simulink model "kalman_estimate_MM"  (R2018b)
settings: Solver=FixedStepAuto  StartTime=0.0  StopTime=500  FixedStep=0.02  RelTol=1e-3
values from neighbouring files (symbols this model uses):
  D = randn(num_output,num_control)    [Com_of_linear_model_calculate.m]    (also in Copy_of_linear_model_calculate.m; D.mat = [0 0 0.00507528406191 0.0236369284061 0.221173094143 0.00198; LINEAR.m = randn(8,1)*10; MM_HKF.m = reshape(out(A_l+B_l+C_l+1:A_l+B_l+C_l+D_l),size_D))
undefined symbols (not defined in the file or in its folder): act_piece, com_piece, piece, sigbuilder_block
libraries: sharedschedule x467, dspsigattribs x44, commchan3 x1
(part 2 of 5)

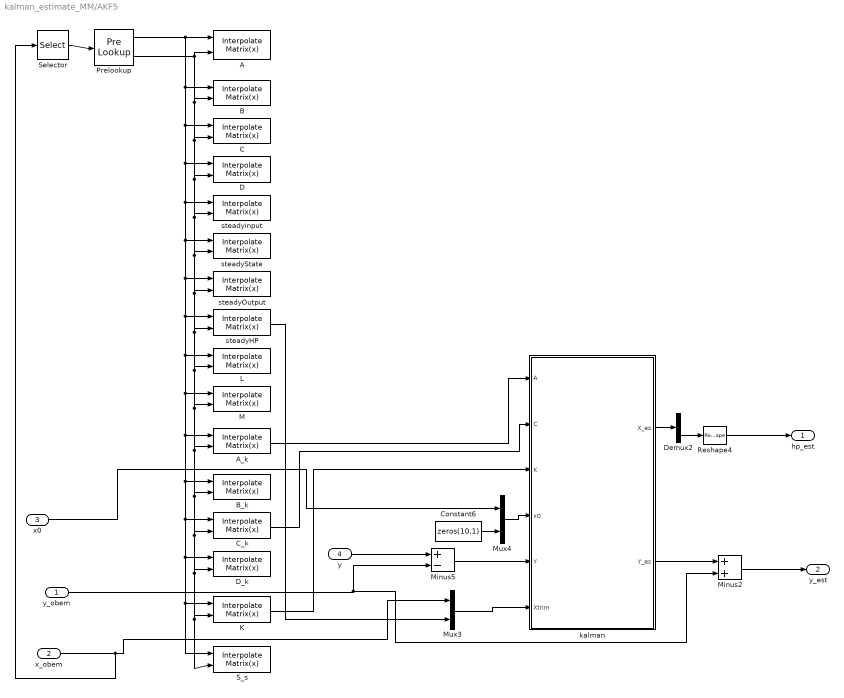
== system kalman_estimate_MM/AKF5 ==
  "y_obem " : Inport
  x_obem : Inport  Port=2
  x0 : Inport  Port=3
  y : Inport  Port=4
  A : sharedschedule/Interpolate Matrix(x)   matrix=piece.A  aMode=aMode
      settings: SourceProductName=Aerospace Blockset  SourceProductBaseCode=AE
  A_k : sharedschedule/Interpolate Matrix(x)   matrix=piece.A_k  aMode=aMode
      settings: SourceProductName=Aerospace Blockset  SourceProductBaseCode=AE
  B : sharedschedule/Interpolate Matrix(x)   matrix=piece.B  aMode=aMode
      settings: SourceProductName=Aerospace Blockset  SourceProductBaseCode=AE
  B_k : sharedschedule/Interpolate Matrix(x)   matrix=piece.B_k  aMode=aMode
      settings: SourceProductName=Aerospace Blockset  SourceProductBaseCode=AE
  C : sharedschedule/Interpolate Matrix(x)   matrix=piece.C  aMode=aMode
      settings: SourceProductName=Aerospace Blockset  SourceProductBaseCode=AE
  C_k : sharedschedule/Interpolate Matrix(x)   matrix=piece.C_k  aMode=aMode
      settings: SourceProductName=Aerospace Blockset  SourceProductBaseCode=AE
  Constant6 : Constant  Value=zeros(10,1)  VectorParams1D=off
  D : sharedschedule/Interpolate Matrix(x)   matrix=piece.D  aMode=aMode
      settings: SourceProductName=Aerospace Blockset  SourceProductBaseCode=AE
  D_k : sharedschedule/Interpolate Matrix(x)   matrix=piece.D_k  aMode=aMode
      settings: SourceProductName=Aerospace Blockset  SourceProductBaseCode=AE
  Demux2 : Demux  Outputs=[2,10]
  K : sharedschedule/Interpolate Matrix(x)   matrix=piece.K  aMode=aMode
      settings: SourceProductName=Aerospace Blockset  SourceProductBaseCode=AE
  L : sharedschedule/Interpolate Matrix(x)   matrix=piece.L  aMode=aMode
      settings: SourceProductName=Aerospace Blockset  SourceProductBaseCode=AE
  M : sharedschedule/Interpolate Matrix(x)   matrix=piece.M  aMode=aMode
      settings: SourceProductName=Aerospace Blockset  SourceProductBaseCode=AE
  Minus2 : Sum
  Minus5 : Sum  Inputs=+-
  Mux3 : Mux  Inputs=2
  Mux4 : Mux  Inputs=2
  Prelookup : PreLookup  BreakpointsData=piece.Nl  BreakpointObject=Nl  ExtrapMethod=Linear  UseLastBreakpoint=on  DiagnosticForOutOfRangeInput=Warning
  Reshape4 : Reshape  OutputDimensionality=Row vector (2-D)
  S_s : sharedschedule/Interpolate Matrix(x)   matrix=piece.K_s  aMode=aMode
      settings: SourceProductName=Aerospace Blockset  SourceProductBaseCode=AE
  Selector : Selector  InputPortWidth=2  IndexOptions=Index vector (dialog)  Indices=[1]  OutputSizes=1
  "kalman " : Subsystem
  steadyHP : sharedschedule/Interpolate Matrix(x)   matrix=piece.steadyHP  aMode=aMode
      settings: SourceProductName=Aerospace Blockset  SourceProductBaseCode=AE
  steadyOutput : sharedschedule/Interpolate Matrix(x)   matrix=piece.steadyOutput  aMode=aMode
      settings: SourceProductName=Aerospace Blockset  SourceProductBaseCode=AE
  steadyState : sharedschedule/Interpolate Matrix(x)   matrix=piece.steadyState  aMode=aMode
      settings: SourceProductName=Aerospace Blockset  SourceProductBaseCode=AE
  steadyinput : sharedschedule/Interpolate Matrix(x)   matrix=piece.steadyInput  aMode=aMode
      settings: SourceProductName=Aerospace Blockset  SourceProductBaseCode=AE
  hp_est : Outport
  y_est : Outport  Port=2
  wires:
  Reshape4/1 -> hp_est/1
  Prelookup/2 -> A/2, S_s/2, K/2, D_k/2, C_k/2, B_k/2, A_k/2, M/2, L/2, steadyHP/2, steadyOutput/2, steadyState/2, steadyinput/2, D/2, C/2, B/2
  Prelookup/1 -> S_s/1, K/1, D_k/1, C_k/1, B_k/1, A_k/1, M/1, L/1, steadyHP/1, steadyOutput/1, steadyState/1, steadyinput/1, D/1, C/1, B/1, A/1
  K/1 -> "kalman "/3(K)
  Selector/1 -> Prelookup/1
  x0/1 -> Mux4/1
  A_k/1 -> "kalman "/1(A)
  "kalman "/1(X_es) -> Demux2/1
  "kalman "/2(Y_es) -> Minus2/1
  Mux3/1 -> "kalman "/6(Xtrim)
  y/1 -> Minus5/1
  Minus5/1 -> "kalman "/5(Y)
  Demux2/2 -> Reshape4/1
  C_k/1 -> "kalman "/2(C)
  "y_obem "/1 -> Minus2/2, Minus5/2
  Mux4/1 -> "kalman "/4(x0)
  Constant6/1 -> Mux4/2
  steadyHP/1 -> Mux3/2
  Minus2/1 -> y_est/1
  x_obem/1 -> Selector/1, Mux3/1

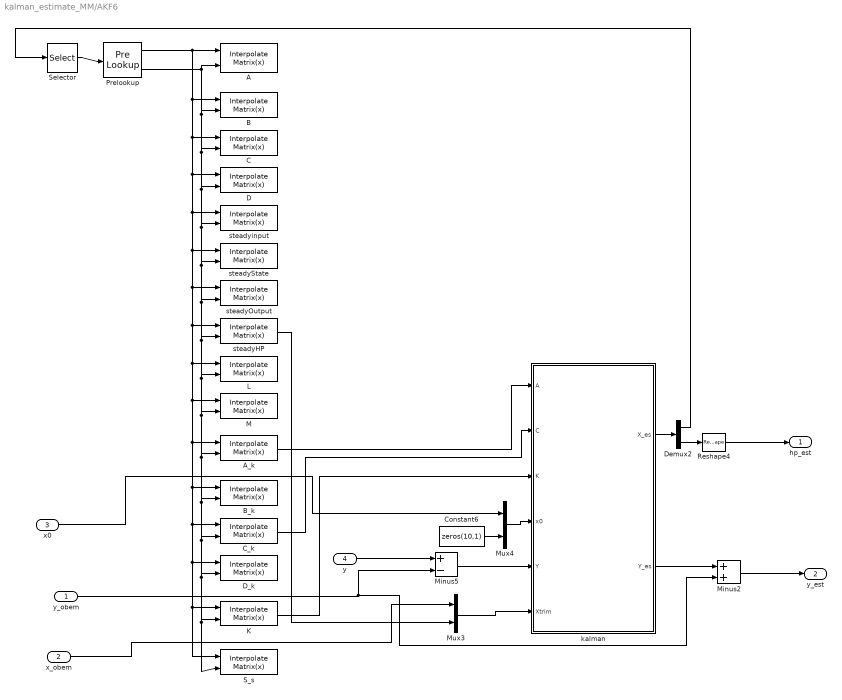
== system kalman_estimate_MM/AKF6 ==
  "y_obem " : Inport
  x_obem : Inport  Port=2
  x0 : Inport  Port=3
  y : Inport  Port=4
  A : sharedschedule/Interpolate Matrix(x)   matrix=piece.A  aMode=aMode
      settings: SourceProductName=Aerospace Blockset  SourceProductBaseCode=AE
  A_k : sharedschedule/Interpolate Matrix(x)   matrix=piece.A_k  aMode=aMode
      settings: SourceProductName=Aerospace Blockset  SourceProductBaseCode=AE
  B : sharedschedule/Interpolate Matrix(x)   matrix=piece.B  aMode=aMode
      settings: SourceProductName=Aerospace Blockset  SourceProductBaseCode=AE
  B_k : sharedschedule/Interpolate Matrix(x)   matrix=piece.B_k  aMode=aMode
      settings: SourceProductName=Aerospace Blockset  SourceProductBaseCode=AE
  C : sharedschedule/Interpolate Matrix(x)   matrix=piece.C  aMode=aMode
      settings: SourceProductName=Aerospace Blockset  SourceProductBaseCode=AE
  C_k : sharedschedule/Interpolate Matrix(x)   matrix=piece.C_k  aMode=aMode
      settings: SourceProductName=Aerospace Blockset  SourceProductBaseCode=AE
  Constant6 : Constant  Value=zeros(10,1)  VectorParams1D=off
  D : sharedschedule/Interpolate Matrix(x)   matrix=piece.D  aMode=aMode
      settings: SourceProductName=Aerospace Blockset  SourceProductBaseCode=AE
  D_k : sharedschedule/Interpolate Matrix(x)   matrix=piece.D_k  aMode=aMode
      settings: SourceProductName=Aerospace Blockset  SourceProductBaseCode=AE
  Demux2 : Demux  Outputs=[2,10]
  K : sharedschedule/Interpolate Matrix(x)   matrix=piece.K  aMode=aMode
      settings: SourceProductName=Aerospace Blockset  SourceProductBaseCode=AE
  L : sharedschedule/Interpolate Matrix(x)   matrix=piece.L  aMode=aMode
      settings: SourceProductName=Aerospace Blockset  SourceProductBaseCode=AE
  M : sharedschedule/Interpolate Matrix(x)   matrix=piece.M  aMode=aMode
      settings: SourceProductName=Aerospace Blockset  SourceProductBaseCode=AE
  Minus2 : Sum
  Minus5 : Sum  Inputs=+-
  Mux3 : Mux  Inputs=2
  Mux4 : Mux  Inputs=2
  Prelookup : PreLookup  BreakpointsData=piece.Nl  BreakpointObject=Nl  ExtrapMethod=Linear  UseLastBreakpoint=on  DiagnosticForOutOfRangeInput=Warning
  Reshape4 : Reshape  OutputDimensionality=Row vector (2-D)
  S_s : sharedschedule/Interpolate Matrix(x)   matrix=piece.K_s  aMode=aMode
      settings: SourceProductName=Aerospace Blockset  SourceProductBaseCode=AE
  Selector : Selector  InputPortWidth=2  IndexOptions=Index vector (dialog)  Indices=[1]  OutputSizes=1
  "kalman " : Subsystem
  steadyHP : sharedschedule/Interpolate Matrix(x)   matrix=piece.steadyHP  aMode=aMode
      settings: SourceProductName=Aerospace Blockset  SourceProductBaseCode=AE
  steadyOutput : sharedschedule/Interpolate Matrix(x)   matrix=piece.steadyOutput  aMode=aMode
      settings: SourceProductName=Aerospace Blockset  SourceProductBaseCode=AE
  steadyState : sharedschedule/Interpolate Matrix(x)   matrix=piece.steadyState  aMode=aMode
      settings: SourceProductName=Aerospace Blockset  SourceProductBaseCode=AE
  steadyinput : sharedschedule/Interpolate Matrix(x)   matrix=piece.steadyInput  aMode=aMode
      settings: SourceProductName=Aerospace Blockset  SourceProductBaseCode=AE
  hp_est : Outport
  y_est : Outport  Port=2
  wires:
  x_obem/1 -> Mux3/1
  Minus2/1 -> y_est/1
  steadyHP/1 -> Mux3/2
  Constant6/1 -> Mux4/2
  Mux4/1 -> "kalman "/4(x0)
  "y_obem "/1 -> Minus5/2, Minus2/2
  C_k/1 -> "kalman "/2(C)
  Demux2/2 -> Reshape4/1
  Minus5/1 -> "kalman "/5(Y)
  y/1 -> Minus5/1
  Mux3/1 -> "kalman "/6(Xtrim)
  "kalman "/2(Y_es) -> Minus2/1
  Demux2/1 -> Selector/1
  "kalman "/1(X_es) -> Demux2/1
  A_k/1 -> "kalman "/1(A)
  x0/1 -> Mux4/1
  Selector/1 -> Prelookup/1
  K/1 -> "kalman "/3(K)
  Prelookup/1 -> A/1, B/1, C/1, D/1, steadyinput/1, steadyState/1, steadyOutput/1, steadyHP/1, L/1, M/1, A_k/1, B_k/1, C_k/1, D_k/1, K/1, S_s/1
  Prelookup/2 -> B/2, C/2, D/2, steadyinput/2, steadyState/2, steadyOutput/2, steadyHP/2, L/2, M/2, A_k/2, B_k/2, C_k/2, D_k/2, K/2, S_s/2, A/2
  Reshape4/1 -> hp_est/1

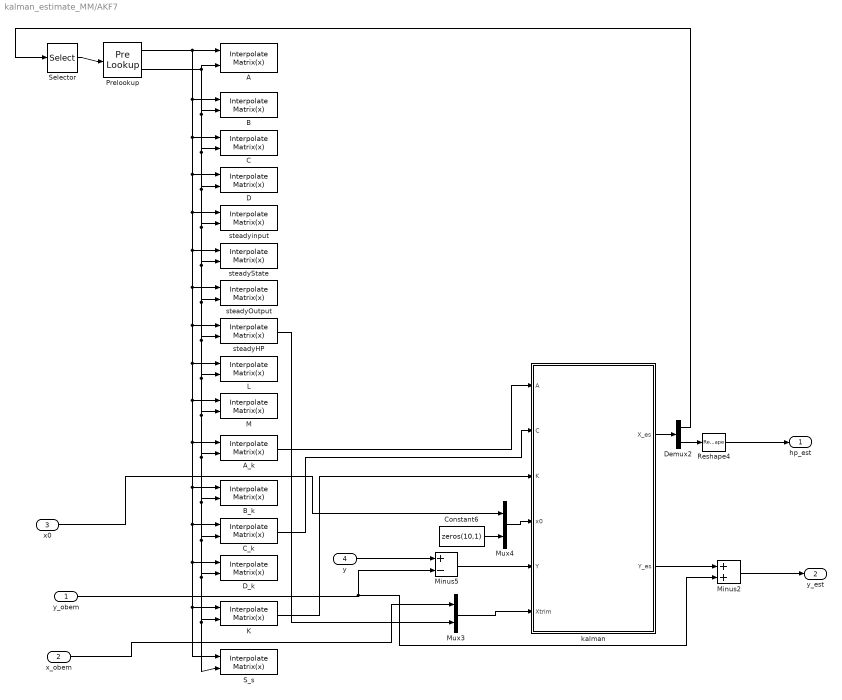
== system kalman_estimate_MM/AKF7 ==
  "y_obem " : Inport
  x_obem : Inport  Port=2
  x0 : Inport  Port=3
  y : Inport  Port=4
  A : sharedschedule/Interpolate Matrix(x)   matrix=piece.A  aMode=aMode
      settings: SourceProductName=Aerospace Blockset  SourceProductBaseCode=AE
  A_k : sharedschedule/Interpolate Matrix(x)   matrix=piece.A_k  aMode=aMode
      settings: SourceProductName=Aerospace Blockset  SourceProductBaseCode=AE
  B : sharedschedule/Interpolate Matrix(x)   matrix=piece.B  aMode=aMode
      settings: SourceProductName=Aerospace Blockset  SourceProductBaseCode=AE
  B_k : sharedschedule/Interpolate Matrix(x)   matrix=piece.B_k  aMode=aMode
      settings: SourceProductName=Aerospace Blockset  SourceProductBaseCode=AE
  C : sharedschedule/Interpolate Matrix(x)   matrix=piece.C  aMode=aMode
      settings: SourceProductName=Aerospace Blockset  SourceProductBaseCode=AE
  C_k : sharedschedule/Interpolate Matrix(x)   matrix=piece.C_k  aMode=aMode
      settings: SourceProductName=Aerospace Blockset  SourceProductBaseCode=AE
  Constant6 : Constant  Value=zeros(10,1)  VectorParams1D=off
  D : sharedschedule/Interpolate Matrix(x)   matrix=piece.D  aMode=aMode
      settings: SourceProductName=Aerospace Blockset  SourceProductBaseCode=AE
  D_k : sharedschedule/Interpolate Matrix(x)   matrix=piece.D_k  aMode=aMode
      settings: SourceProductName=Aerospace Blockset  SourceProductBaseCode=AE
  Demux2 : Demux  Outputs=[2,10]
  K : sharedschedule/Interpolate Matrix(x)   matrix=piece.K  aMode=aMode
      settings: SourceProductName=Aerospace Blockset  SourceProductBaseCode=AE
  L : sharedschedule/Interpolate Matrix(x)   matrix=piece.L  aMode=aMode
      settings: SourceProductName=Aerospace Blockset  SourceProductBaseCode=AE
  M : sharedschedule/Interpolate Matrix(x)   matrix=piece.M  aMode=aMode
      settings: SourceProductName=Aerospace Blockset  SourceProductBaseCode=AE
  Minus2 : Sum
  Minus5 : Sum  Inputs=+-
  Mux3 : Mux  Inputs=2
  Mux4 : Mux  Inputs=2
  Prelookup : PreLookup  BreakpointsData=piece.Nl  BreakpointObject=Nl  ExtrapMethod=Linear  UseLastBreakpoint=on  DiagnosticForOutOfRangeInput=Warning
  Reshape4 : Reshape  OutputDimensionality=Row vector (2-D)
  S_s : sharedschedule/Interpolate Matrix(x)   matrix=piece.K_s  aMode=aMode
      settings: SourceProductName=Aerospace Blockset  SourceProductBaseCode=AE
  Selector : Selector  InputPortWidth=2  IndexOptions=Index vector (dialog)  Indices=[1]  OutputSizes=1
  "kalman " : Subsystem
  steadyHP : sharedschedule/Interpolate Matrix(x)   matrix=piece.steadyHP  aMode=aMode
      settings: SourceProductName=Aerospace Blockset  SourceProductBaseCode=AE
  steadyOutput : sharedschedule/Interpolate Matrix(x)   matrix=piece.steadyOutput  aMode=aMode
      settings: SourceProductName=Aerospace Blockset  SourceProductBaseCode=AE
  steadyState : sharedschedule/Interpolate Matrix(x)   matrix=piece.steadyState  aMode=aMode
      settings: SourceProductName=Aerospace Blockset  SourceProductBaseCode=AE
  steadyinput : sharedschedule/Interpolate Matrix(x)   matrix=piece.steadyInput  aMode=aMode
      settings: SourceProductName=Aerospace Blockset  SourceProductBaseCode=AE
  hp_est : Outport
  y_est : Outport  Port=2
  wires:
  Reshape4/1 -> hp_est/1
  Prelookup/2 -> A/2, S_s/2, K/2, D_k/2, C_k/2, B_k/2, A_k/2, M/2, L/2, steadyHP/2, steadyOutput/2, steadyState/2, steadyinput/2, D/2, C/2, B/2
  Prelookup/1 -> S_s/1, K/1, D_k/1, C_k/1, B_k/1, A_k/1, M/1, L/1, steadyHP/1, steadyOutput/1, steadyState/1, steadyinput/1, D/1, C/1, B/1, A/1
  K/1 -> "kalman "/3(K)
  Selector/1 -> Prelookup/1
  x0/1 -> Mux4/1
  A_k/1 -> "kalman "/1(A)
  "kalman "/1(X_es) -> Demux2/1
  Demux2/1 -> Selector/1
  "kalman "/2(Y_es) -> Minus2/1
  Mux3/1 -> "kalman "/6(Xtrim)
  y/1 -> Minus5/1
  Minus5/1 -> "kalman "/5(Y)
  Demux2/2 -> Reshape4/1
  C_k/1 -> "kalman "/2(C)
  "y_obem "/1 -> Minus2/2, Minus5/2
  Mux4/1 -> "kalman "/4(x0)
  Constant6/1 -> Mux4/2
  steadyHP/1 -> Mux3/2
  Minus2/1 -> y_est/1
  x_obem/1 -> Mux3/1

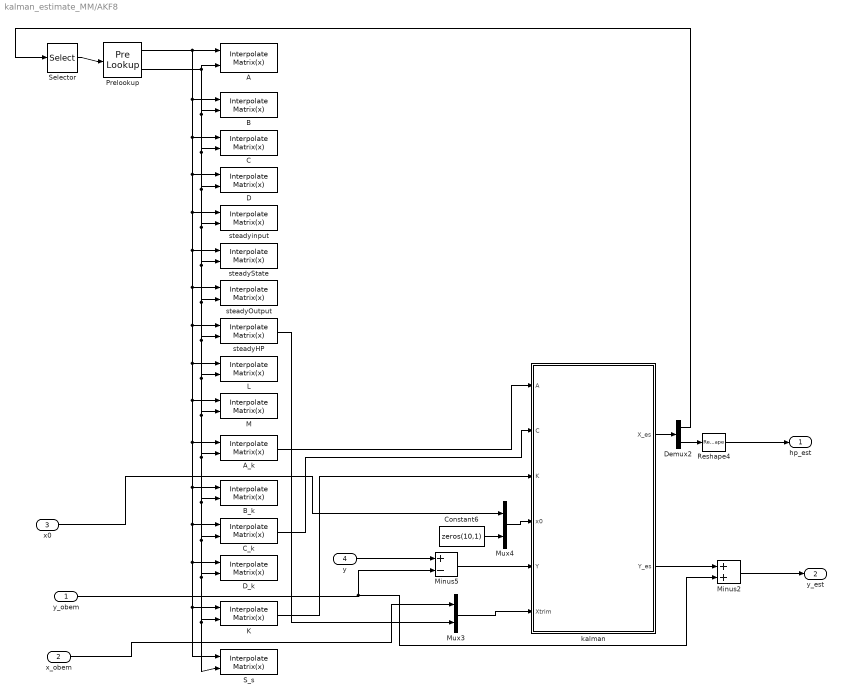
== system kalman_estimate_MM/AKF8 ==
  "y_obem " : Inport
  x_obem : Inport  Port=2
  x0 : Inport  Port=3
  y : Inport  Port=4
  A : sharedschedule/Interpolate Matrix(x)   matrix=piece.A  aMode=aMode
      settings: SourceProductName=Aerospace Blockset  SourceProductBaseCode=AE
  A_k : sharedschedule/Interpolate Matrix(x)   matrix=piece.A_k  aMode=aMode
      settings: SourceProductName=Aerospace Blockset  SourceProductBaseCode=AE
  B : sharedschedule/Interpolate Matrix(x)   matrix=piece.B  aMode=aMode
      settings: SourceProductName=Aerospace Blockset  SourceProductBaseCode=AE
  B_k : sharedschedule/Interpolate Matrix(x)   matrix=piece.B_k  aMode=aMode
      settings: SourceProductName=Aerospace Blockset  SourceProductBaseCode=AE
  C : sharedschedule/Interpolate Matrix(x)   matrix=piece.C  aMode=aMode
      settings: SourceProductName=Aerospace Blockset  SourceProductBaseCode=AE
  C_k : sharedschedule/Interpolate Matrix(x)   matrix=piece.C_k  aMode=aMode
      settings: SourceProductName=Aerospace Blockset  SourceProductBaseCode=AE
  Constant6 : Constant  Value=zeros(10,1)  VectorParams1D=off
  D : sharedschedule/Interpolate Matrix(x)   matrix=piece.D  aMode=aMode
      settings: SourceProductName=Aerospace Blockset  SourceProductBaseCode=AE
  D_k : sharedschedule/Interpolate Matrix(x)   matrix=piece.D_k  aMode=aMode
      settings: SourceProductName=Aerospace Blockset  SourceProductBaseCode=AE
  Demux2 : Demux  Outputs=[2,10]
  K : sharedschedule/Interpolate Matrix(x)   matrix=piece.K  aMode=aMode
      settings: SourceProductName=Aerospace Blockset  SourceProductBaseCode=AE
  L : sharedschedule/Interpolate Matrix(x)   matrix=piece.L  aMode=aMode
      settings: SourceProductName=Aerospace Blockset  SourceProductBaseCode=AE
  M : sharedschedule/Interpolate Matrix(x)   matrix=piece.M  aMode=aMode
      settings: SourceProductName=Aerospace Blockset  SourceProductBaseCode=AE
  Minus2 : Sum
  Minus5 : Sum  Inputs=+-
  Mux3 : Mux  Inputs=2
  Mux4 : Mux  Inputs=2
  Prelookup : PreLookup  BreakpointsData=piece.Nl  BreakpointObject=Nl  ExtrapMethod=Linear  UseLastBreakpoint=on  DiagnosticForOutOfRangeInput=Warning
  Reshape4 : Reshape  OutputDimensionality=Row vector (2-D)
  S_s : sharedschedule/Interpolate Matrix(x)   matrix=piece.K_s  aMode=aMode
      settings: SourceProductName=Aerospace Blockset  SourceProductBaseCode=AE
  Selector : Selector  InputPortWidth=2  IndexOptions=Index vector (dialog)  Indices=[1]  OutputSizes=1
  "kalman " : Subsystem
  steadyHP : sharedschedule/Interpolate Matrix(x)   matrix=piece.steadyHP  aMode=aMode
      settings: SourceProductName=Aerospace Blockset  SourceProductBaseCode=AE
  steadyOutput : sharedschedule/Interpolate Matrix(x)   matrix=piece.steadyOutput  aMode=aMode
      settings: SourceProductName=Aerospace Blockset  SourceProductBaseCode=AE
  steadyState : sharedschedule/Interpolate Matrix(x)   matrix=piece.steadyState  aMode=aMode
      settings: SourceProductName=Aerospace Blockset  SourceProductBaseCode=AE
  steadyinput : sharedschedule/Interpolate Matrix(x)   matrix=piece.steadyInput  aMode=aMode
      settings: SourceProductName=Aerospace Blockset  SourceProductBaseCode=AE
  hp_est : Outport
  y_est : Outport  Port=2
  wires:
  x_obem/1 -> Mux3/1
  Minus2/1 -> y_est/1
  steadyHP/1 -> Mux3/2
  Constant6/1 -> Mux4/2
  Mux4/1 -> "kalman "/4(x0)
  "y_obem "/1 -> Minus5/2, Minus2/2
  C_k/1 -> "kalman "/2(C)
  Demux2/2 -> Reshape4/1
  Minus5/1 -> "kalman "/5(Y)
  y/1 -> Minus5/1
  Mux3/1 -> "kalman "/6(Xtrim)
  "kalman "/2(Y_es) -> Minus2/1
  Demux2/1 -> Selector/1
  "kalman "/1(X_es) -> Demux2/1
  A_k/1 -> "kalman "/1(A)
  x0/1 -> Mux4/1
  Selector/1 -> Prelookup/1
  K/1 -> "kalman "/3(K)
  Prelookup/1 -> A/1, B/1, C/1, D/1, steadyinput/1, steadyState/1, steadyOutput/1, steadyHP/1, L/1, M/1, A_k/1, B_k/1, C_k/1, D_k/1, K/1, S_s/1
  Prelookup/2 -> B/2, C/2, D/2, steadyinput/2, steadyState/2, steadyOutput/2, steadyHP/2, L/2, M/2, A_k/2, B_k/2, C_k/2, D_k/2, K/2, S_s/2, A/2
  Reshape4/1 -> hp_est/1

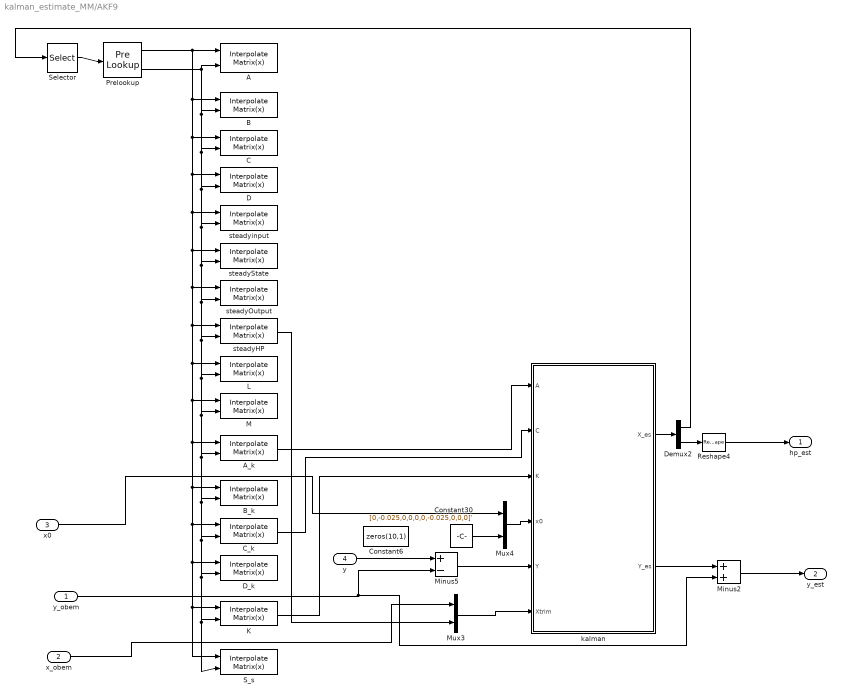
== system kalman_estimate_MM/AKF9 ==
  "y_obem " : Inport
  x_obem : Inport  Port=2
  x0 : Inport  Port=3
  y : Inport  Port=4
  A : sharedschedule/Interpolate Matrix(x)   matrix=piece.A  aMode=aMode
      settings: SourceProductName=Aerospace Blockset  SourceProductBaseCode=AE
  A_k : sharedschedule/Interpolate Matrix(x)   matrix=piece.A_k  aMode=aMode
      settings: SourceProductName=Aerospace Blockset  SourceProductBaseCode=AE
  B : sharedschedule/Interpolate Matrix(x)   matrix=piece.B  aMode=aMode
      settings: SourceProductName=Aerospace Blockset  SourceProductBaseCode=AE
  B_k : sharedschedule/Interpolate Matrix(x)   matrix=piece.B_k  aMode=aMode
      settings: SourceProductName=Aerospace Blockset  SourceProductBaseCode=AE
  C : sharedschedule/Interpolate Matrix(x)   matrix=piece.C  aMode=aMode
      settings: SourceProductName=Aerospace Blockset  SourceProductBaseCode=AE
  C_k : sharedschedule/Interpolate Matrix(x)   matrix=piece.C_k  aMode=aMode
      settings: SourceProductName=Aerospace Blockset  SourceProductBaseCode=AE
  Constant30 : Constant  Value=[0,-0.025,0,0,0,0,-0.025,0,0,0]'  VectorParams1D=off
  Constant6 : Constant  Value=zeros(10,1)  VectorParams1D=off
  D : sharedschedule/Interpolate Matrix(x)   matrix=piece.D  aMode=aMode
      settings: SourceProductName=Aerospace Blockset  SourceProductBaseCode=AE
  D_k : sharedschedule/Interpolate Matrix(x)   matrix=piece.D_k  aMode=aMode
      settings: SourceProductName=Aerospace Blockset  SourceProductBaseCode=AE
  Demux2 : Demux  Outputs=[2,10]
  K : sharedschedule/Interpolate Matrix(x)   matrix=piece.K  aMode=aMode
      settings: SourceProductName=Aerospace Blockset  SourceProductBaseCode=AE
  L : sharedschedule/Interpolate Matrix(x)   matrix=piece.L  aMode=aMode
      settings: SourceProductName=Aerospace Blockset  SourceProductBaseCode=AE
  M : sharedschedule/Interpolate Matrix(x)   matrix=piece.M  aMode=aMode
      settings: SourceProductName=Aerospace Blockset  SourceProductBaseCode=AE
  Minus2 : Sum
  Minus5 : Sum  Inputs=+-
  Mux3 : Mux  Inputs=2
  Mux4 : Mux  Inputs=2
  Prelookup : PreLookup  BreakpointsData=piece.Nl  BreakpointObject=Nl  ExtrapMethod=Linear  UseLastBreakpoint=on  DiagnosticForOutOfRangeInput=Warning
  Reshape4 : Reshape  OutputDimensionality=Row vector (2-D)
  S_s : sharedschedule/Interpolate Matrix(x)   matrix=piece.K_s  aMode=aMode
      settings: SourceProductName=Aerospace Blockset  SourceProductBaseCode=AE
  Selector : Selector  InputPortWidth=2  IndexOptions=Index vector (dialog)  Indices=[1]  OutputSizes=1
  "kalman " : Subsystem
  steadyHP : sharedschedule/Interpolate Matrix(x)   matrix=piece.steadyHP  aMode=aMode
      settings: SourceProductName=Aerospace Blockset  SourceProductBaseCode=AE
  steadyOutput : sharedschedule/Interpolate Matrix(x)   matrix=piece.steadyOutput  aMode=aMode
      settings: SourceProductName=Aerospace Blockset  SourceProductBaseCode=AE
  steadyState : sharedschedule/Interpolate Matrix(x)   matrix=piece.steadyState  aMode=aMode
      settings: SourceProductName=Aerospace Blockset  SourceProductBaseCode=AE
  steadyinput : sharedschedule/Interpolate Matrix(x)   matrix=piece.steadyInput  aMode=aMode
      settings: SourceProductName=Aerospace Blockset  SourceProductBaseCode=AE
  hp_est : Outport
  y_est : Outport  Port=2
  wires:
  Reshape4/1 -> hp_est/1
  Prelookup/2 -> A/2, S_s/2, K/2, D_k/2, C_k/2, B_k/2, A_k/2, M/2, L/2, steadyHP/2, steadyOutput/2, steadyState/2, steadyinput/2, D/2, C/2, B/2
  Prelookup/1 -> S_s/1, K/1, D_k/1, C_k/1, B_k/1, A_k/1, M/1, L/1, steadyHP/1, steadyOutput/1, steadyState/1, steadyinput/1, D/1, C/1, B/1, A/1
  K/1 -> "kalman "/3(K)
  Selector/1 -> Prelookup/1
  x0/1 -> Mux4/1
  A_k/1 -> "kalman "/1(A)
  "kalman "/1(X_es) -> Demux2/1
  Demux2/1 -> Selector/1
  "kalman "/2(Y_es) -> Minus2/1
  Mux3/1 -> "kalman "/6(Xtrim)
  y/1 -> Minus5/1
  Minus5/1 -> "kalman "/5(Y)
  Demux2/2 -> Reshape4/1
  C_k/1 -> "kalman "/2(C)
  "y_obem "/1 -> Minus2/2, Minus5/2
  Mux4/1 -> "kalman "/4(x0)
  steadyHP/1 -> Mux3/2
  Minus2/1 -> y_est/1
  x_obem/1 -> Mux3/1
  Constant30/1 -> Mux4/2

== system kalman_estimate_MM/HKF1 ==
  In2 : Inport
  In3 : Inport  Port=2
  In4 : Inport  Port=3
  x_obem : Inport  Port=4
  y_obem : Inport  Port=5
  A : sharedschedule/Interpolate Matrix(x)   matrix=piece.A  aMode=aMode
      settings: SourceProductName=Aerospace Blockset  SourceProductBaseCode=AE
  B : sharedschedule/Interpolate Matrix(x)   matrix=piece.B  aMode=aMode
      settings: SourceProductName=Aerospace Blockset  SourceProductBaseCode=AE
  C : sharedschedule/Interpolate Matrix(x)   matrix=piece.C  aMode=aMode
      settings: SourceProductName=Aerospace Blockset  SourceProductBaseCode=AE
  D : sharedschedule/Interpolate Matrix(x)   matrix=piece.D  aMode=aMode
      settings: SourceProductName=Aerospace Blockset  SourceProductBaseCode=AE
  K_s : sharedschedule/Interpolate Matrix(x)   matrix=piece.K_s  aMode=aMode
      settings: SourceProductName=Aerospace Blockset  SourceProductBaseCode=AE
  L : sharedschedule/Interpolate Matrix(x)   matrix=piece.L  aMode=aMode
      settings: SourceProductName=Aerospace Blockset  SourceProductBaseCode=AE
  M : sharedschedule/Interpolate Matrix(x)   matrix=piece.M  aMode=aMode
      settings: SourceProductName=Aerospace Blockset  SourceProductBaseCode=AE
  MATLAB Function : MATLAB Function  TreatAsAtomicUnit=on
  Minus5 : Sum  Inputs=+-
  Prelookup : PreLookup  BreakpointsData=piece.Nl  BreakpointObject=Nl  ExtrapMethod=Linear  UseLastBreakpoint=on  DiagnosticForOutOfRangeInput=Warning
  S : sharedschedule/Interpolate Matrix(x)   matrix=piece.S_s  aMode=aMode
      settings: SourceProductName=Aerospace Blockset  SourceProductBaseCode=AE
  Selector : Selector  InputPortWidth=2  IndexOptions=Index vector (dialog)  Indices=[1]  OutputSizes=1
  kalman filter1 : Subsystem
  steadyOutput : sharedschedule/Interpolate Matrix(x)   matrix=piece.steadyOutput  aMode=aMode
      settings: SourceProductName=Aerospace Blockset  SourceProductBaseCode=AE
  steadyState : sharedschedule/Interpolate Matrix(x)   matrix=piece.steadyState  aMode=aMode
      settings: SourceProductName=Aerospace Blockset  SourceProductBaseCode=AE
  steadyinput : sharedschedule/Interpolate Matrix(x)   matrix=piece.steadyInput  aMode=aMode
      settings: SourceProductName=Aerospace Blockset  SourceProductBaseCode=AE
  Out1 : Outport
  Out2 : Outport  Port=2
  Out3 : Outport  Port=3
  wires:
  x_obem/1 -> kalman filter1/6(Xtrim)
  y_obem/1 -> Minus5/2
  In2/1 -> Minus5/1
  In3/1 -> kalman filter1/4(x0)
  M/1 -> kalman filter1/8(M)
  A/1 -> kalman filter1/1(A)
  K_s/1 -> kalman filter1/3(K)
  kalman filter1/1(X_es) -> Selector/1
  kalman filter1/2(Y_es) -> Out1/1
  Minus5/1 -> kalman filter1/5(Y)
  C/1 -> kalman filter1/2(C)
  L/1 -> kalman filter1/7(L)
  Selector/1 -> Prelookup/1
  Prelookup/2 -> B/2, C/2, D/2, steadyOutput/2, steadyinput/2, L/2, M/2, K_s/2, S/2, steadyState/2, A/2
  In4/1 -> kalman filter1/9(P)
  Prelookup/1 -> A/1, B/1, C/1, D/1, steadyOutput/1, steadyinput/1, steadyState/1, L/1, M/1, K_s/1, S/1
  MATLAB Function/1(y) -> Out3/1
  kalman filter1/3(Y_error) -> MATLAB Function/1(err), Out2/1
  S/1 -> MATLAB Function/2(S)

== system kalman_estimate_MM/HKF10 ==
  In3 : Inport
  In4 : Inport  Port=2
  x_obem : Inport  Port=3
  y_obem : Inport  Port=4
  A : sharedschedule/Interpolate Matrix(x)   matrix=piece.A  aMode=aMode
      settings: SourceProductName=Aerospace Blockset  SourceProductBaseCode=AE
  Add : Sum
  B : sharedschedule/Interpolate Matrix(x)   matrix=piece.B  aMode=aMode
      settings: SourceProductName=Aerospace Blockset  SourceProductBaseCode=AE
  C : sharedschedule/Interpolate Matrix(x)   matrix=piece.C  aMode=aMode
      settings: SourceProductName=Aerospace Blockset  SourceProductBaseCode=AE
  D : sharedschedule/Interpolate Matrix(x)   matrix=piece.D  aMode=aMode
      settings: SourceProductName=Aerospace Blockset  SourceProductBaseCode=AE
  K_s : sharedschedule/Interpolate Matrix(x)   matrix=piece.K_s  aMode=aMode
      settings: SourceProductName=Aerospace Blockset  SourceProductBaseCode=AE
  L : sharedschedule/Interpolate Matrix(x)   matrix=piece.L  aMode=aMode
      settings: SourceProductName=Aerospace Blockset  SourceProductBaseCode=AE
  M : sharedschedule/Interpolate Matrix(x)   matrix=piece.M  aMode=aMode
      settings: SourceProductName=Aerospace Blockset  SourceProductBaseCode=AE
  Prelookup : PreLookup  BreakpointsData=piece.Nl  BreakpointObject=Nl  ExtrapMethod=Linear  UseLastBreakpoint=on  DiagnosticForOutOfRangeInput=Warning
  S : sharedschedule/Interpolate Matrix(x)   matrix=piece.S_s  aMode=aMode
      settings: SourceProductName=Aerospace Blockset  SourceProductBaseCode=AE
  Selector : Selector  InputPortWidth=2  IndexOptions=Index vector (dialog)  Indices=[1]  OutputSizes=1
  kalman filter1 : Subsystem
  steadyOutput : sharedschedule/Interpolate Matrix(x)   matrix=piece.steadyOutput  aMode=aMode
      settings: SourceProductName=Aerospace Blockset  SourceProductBaseCode=AE
  steadyState : sharedschedule/Interpolate Matrix(x)   matrix=piece.steadyState  aMode=aMode
      settings: SourceProductName=Aerospace Blockset  SourceProductBaseCode=AE
  steadyinput : sharedschedule/Interpolate Matrix(x)   matrix=piece.steadyInput  aMode=aMode
      settings: SourceProductName=Aerospace Blockset  SourceProductBaseCode=AE
  Out1 : Outport
  Out2 : Outport  Port=2
  wires:
  Prelookup/1 -> S/1, K_s/1, M/1, L/1, steadyState/1, steadyinput/1, steadyOutput/1, D/1, C/1, B/1, A/1
  In4/1 -> kalman filter1/7(P)
  Prelookup/2 -> A/2, steadyState/2, S/2, K_s/2, M/2, L/2, steadyinput/2, steadyOutput/2, D/2, C/2, B/2
  Selector/1 -> Prelookup/1
  L/1 -> kalman filter1/5(L)
  C/1 -> kalman filter1/2(C)
  kalman filter1/1(X_es) -> Selector/1
  A/1 -> kalman filter1/1(A)
  M/1 -> kalman filter1/6(M)
  In3/1 -> kalman filter1/3(x0)
  x_obem/1 -> kalman filter1/4(Xtrim)
  y_obem/1 -> Add/2
  kalman filter1/2(Y_es) -> Add/1, Out1/1
  Add/1 -> Out2/1

== system kalman_estimate_MM/HKF11 ==
  In3 : Inport
  In4 : Inport  Port=2
  x_obem : Inport  Port=3
  y_obem : Inport  Port=4
  A : sharedschedule/Interpolate Matrix(x)   matrix=piece.A  aMode=aMode
      settings: SourceProductName=Aerospace Blockset  SourceProductBaseCode=AE
  Add : Sum
  B : sharedschedule/Interpolate Matrix(x)   matrix=piece.B  aMode=aMode
      settings: SourceProductName=Aerospace Blockset  SourceProductBaseCode=AE
  C : sharedschedule/Interpolate Matrix(x)   matrix=piece.C  aMode=aMode
      settings: SourceProductName=Aerospace Blockset  SourceProductBaseCode=AE
  D : sharedschedule/Interpolate Matrix(x)   matrix=piece.D  aMode=aMode
      settings: SourceProductName=Aerospace Blockset  SourceProductBaseCode=AE
  K_s : sharedschedule/Interpolate Matrix(x)   matrix=piece.K_s  aMode=aMode
      settings: SourceProductName=Aerospace Blockset  SourceProductBaseCode=AE
  L : sharedschedule/Interpolate Matrix(x)   matrix=piece.L  aMode=aMode
      settings: SourceProductName=Aerospace Blockset  SourceProductBaseCode=AE
  M : sharedschedule/Interpolate Matrix(x)   matrix=piece.M  aMode=aMode
      settings: SourceProductName=Aerospace Blockset  SourceProductBaseCode=AE
  Prelookup : PreLookup  BreakpointsData=piece.Nl  BreakpointObject=Nl  ExtrapMethod=Linear  UseLastBreakpoint=on  DiagnosticForOutOfRangeInput=Warning
  S : sharedschedule/Interpolate Matrix(x)   matrix=piece.S_s  aMode=aMode
      settings: SourceProductName=Aerospace Blockset  SourceProductBaseCode=AE
  Selector : Selector  InputPortWidth=2  IndexOptions=Index vector (dialog)  Indices=[1]  OutputSizes=1
  kalman filter1 : Subsystem
  steadyOutput : sharedschedule/Interpolate Matrix(x)   matrix=piece.steadyOutput  aMode=aMode
      settings: SourceProductName=Aerospace Blockset  SourceProductBaseCode=AE
  steadyState : sharedschedule/Interpolate Matrix(x)   matrix=piece.steadyState  aMode=aMode
      settings: SourceProductName=Aerospace Blockset  SourceProductBaseCode=AE
  steadyinput : sharedschedule/Interpolate Matrix(x)   matrix=piece.steadyInput  aMode=aMode
      settings: SourceProductName=Aerospace Blockset  SourceProductBaseCode=AE
  Out1 : Outport
  Out2 : Outport  Port=2
  wires:
  Add/1 -> Out2/1
  kalman filter1/2(Y_es) -> Out1/1, Add/1
  y_obem/1 -> Add/2
  x_obem/1 -> kalman filter1/4(Xtrim)
  In3/1 -> kalman filter1/3(x0)
  M/1 -> kalman filter1/6(M)
  A/1 -> kalman filter1/1(A)
  kalman filter1/1(X_es) -> Selector/1
  C/1 -> kalman filter1/2(C)
  L/1 -> kalman filter1/5(L)
  Selector/1 -> Prelookup/1
  Prelookup/2 -> B/2, C/2, D/2, steadyOutput/2, steadyinput/2, L/2, M/2, K_s/2, S/2, steadyState/2, A/2
  In4/1 -> kalman filter1/7(P)
  Prelookup/1 -> A/1, B/1, C/1, D/1, steadyOutput/1, steadyinput/1, steadyState/1, L/1, M/1, K_s/1, S/1

== system kalman_estimate_MM/HKF2 ==
  In3 : Inport
  In4 : Inport  Port=2
  x_obem : Inport  Port=3
  y_obem : Inport  Port=4
  A : sharedschedule/Interpolate Matrix(x)   matrix=piece.A  aMode=aMode
      settings: SourceProductName=Aerospace Blockset  SourceProductBaseCode=AE
  Add : Sum
  B : sharedschedule/Interpolate Matrix(x)   matrix=piece.B  aMode=aMode
      settings: SourceProductName=Aerospace Blockset  SourceProductBaseCode=AE
  C : sharedschedule/Interpolate Matrix(x)   matrix=piece.C  aMode=aMode
      settings: SourceProductName=Aerospace Blockset  SourceProductBaseCode=AE
  D : sharedschedule/Interpolate Matrix(x)   matrix=piece.D  aMode=aMode
      settings: SourceProductName=Aerospace Blockset  SourceProductBaseCode=AE
  K_s : sharedschedule/Interpolate Matrix(x)   matrix=piece.K_s  aMode=aMode
      settings: SourceProductName=Aerospace Blockset  SourceProductBaseCode=AE
  L : sharedschedule/Interpolate Matrix(x)   matrix=piece.L  aMode=aMode
      settings: SourceProductName=Aerospace Blockset  SourceProductBaseCode=AE
  M : sharedschedule/Interpolate Matrix(x)   matrix=piece.M  aMode=aMode
      settings: SourceProductName=Aerospace Blockset  SourceProductBaseCode=AE
  Prelookup : PreLookup  BreakpointsData=piece.Nl  BreakpointObject=Nl  ExtrapMethod=Linear  UseLastBreakpoint=on  DiagnosticForOutOfRangeInput=Warning
  S : sharedschedule/Interpolate Matrix(x)   matrix=piece.S_s  aMode=aMode
      settings: SourceProductName=Aerospace Blockset  SourceProductBaseCode=AE
  Selector : Selector  InputPortWidth=2  IndexOptions=Index vector (dialog)  Indices=[1]  OutputSizes=1
  kalman filter1 : Subsystem
  steadyOutput : sharedschedule/Interpolate Matrix(x)   matrix=piece.steadyOutput  aMode=aMode
      settings: SourceProductName=Aerospace Blockset  SourceProductBaseCode=AE
  steadyState : sharedschedule/Interpolate Matrix(x)   matrix=piece.steadyState  aMode=aMode
      settings: SourceProductName=Aerospace Blockset  SourceProductBaseCode=AE
  steadyinput : sharedschedule/Interpolate Matrix(x)   matrix=piece.steadyInput  aMode=aMode
      settings: SourceProductName=Aerospace Blockset  SourceProductBaseCode=AE
  Out1 : Outport
  Out2 : Outport  Port=2
  wires:
  Add/1 -> Out2/1
  kalman filter1/2(Y_es) -> Out1/1, Add/1
  y_obem/1 -> Add/2
  x_obem/1 -> kalman filter1/4(Xtrim)
  In3/1 -> kalman filter1/3(x0)
  M/1 -> kalman filter1/6(M)
  A/1 -> kalman filter1/1(A)
  kalman filter1/1(X_es) -> Selector/1
  C/1 -> kalman filter1/2(C)
  L/1 -> kalman filter1/5(L)
  Selector/1 -> Prelookup/1
  Prelookup/2 -> B/2, C/2, D/2, steadyOutput/2, steadyinput/2, L/2, M/2, K_s/2, S/2, steadyState/2, A/2
  In4/1 -> kalman filter1/7(P)
  Prelookup/1 -> A/1, B/1, C/1, D/1, steadyOutput/1, steadyinput/1, steadyState/1, L/1, M/1, K_s/1, S/1

== system kalman_estimate_MM/HKF3 ==
  In2 : Inport
  In3 : Inport  Port=2
  In4 : Inport  Port=3
  x_obem : Inport  Port=4
  y_obem : Inport  Port=5
  A : sharedschedule/Interpolate Matrix(x)   matrix=piece.A  aMode=aMode
      settings: SourceProductName=Aerospace Blockset  SourceProductBaseCode=AE
  B : sharedschedule/Interpolate Matrix(x)   matrix=piece.B  aMode=aMode
      settings: SourceProductName=Aerospace Blockset  SourceProductBaseCode=AE
  C : sharedschedule/Interpolate Matrix(x)   matrix=piece.C  aMode=aMode
      settings: SourceProductName=Aerospace Blockset  SourceProductBaseCode=AE
  D : sharedschedule/Interpolate Matrix(x)   matrix=piece.D  aMode=aMode
      settings: SourceProductName=Aerospace Blockset  SourceProductBaseCode=AE
  K_s : sharedschedule/Interpolate Matrix(x)   matrix=piece.K_s  aMode=aMode
      settings: SourceProductName=Aerospace Blockset  SourceProductBaseCode=AE
  L : sharedschedule/Interpolate Matrix(x)   matrix=piece.L  aMode=aMode
      settings: SourceProductName=Aerospace Blockset  SourceProductBaseCode=AE
  M : sharedschedule/Interpolate Matrix(x)   matrix=piece.M  aMode=aMode
      settings: SourceProductName=Aerospace Blockset  SourceProductBaseCode=AE
  MATLAB Function : MATLAB Function  TreatAsAtomicUnit=on
  Minus5 : Sum  Inputs=+-
  Prelookup : PreLookup  BreakpointsData=piece.Nl  BreakpointObject=Nl  ExtrapMethod=Linear  UseLastBreakpoint=on  DiagnosticForOutOfRangeInput=Warning
  S : sharedschedule/Interpolate Matrix(x)   matrix=piece.S_s  aMode=aMode
      settings: SourceProductName=Aerospace Blockset  SourceProductBaseCode=AE
  Selector : Selector  InputPortWidth=2  IndexOptions=Index vector (dialog)  Indices=[1]  OutputSizes=1
  kalman filter1 : Subsystem
  steadyOutput : sharedschedule/Interpolate Matrix(x)   matrix=piece.steadyOutput  aMode=aMode
      settings: SourceProductName=Aerospace Blockset  SourceProductBaseCode=AE
  steadyState : sharedschedule/Interpolate Matrix(x)   matrix=piece.steadyState  aMode=aMode
      settings: SourceProductName=Aerospace Blockset  SourceProductBaseCode=AE
  steadyinput : sharedschedule/Interpolate Matrix(x)   matrix=piece.steadyInput  aMode=aMode
      settings: SourceProductName=Aerospace Blockset  SourceProductBaseCode=AE
  Out1 : Outport
  Out2 : Outport  Port=2
  Out3 : Outport  Port=3
  wires:
  x_obem/1 -> kalman filter1/6(Xtrim)
  y_obem/1 -> Minus5/2
  In2/1 -> Minus5/1
  In3/1 -> kalman filter1/4(x0)
  M/1 -> kalman filter1/8(M)
  A/1 -> kalman filter1/1(A)
  K_s/1 -> kalman filter1/3(K)
  kalman filter1/1(X_es) -> Selector/1
  kalman filter1/2(Y_es) -> Out1/1
  Minus5/1 -> kalman filter1/5(Y)
  C/1 -> kalman filter1/2(C)
  L/1 -> kalman filter1/7(L)
  Selector/1 -> Prelookup/1
  Prelookup/2 -> B/2, C/2, D/2, steadyOutput/2, steadyinput/2, L/2, M/2, K_s/2, S/2, steadyState/2, A/2
  In4/1 -> kalman filter1/9(P)
  Prelookup/1 -> A/1, B/1, C/1, D/1, steadyOutput/1, steadyinput/1, steadyState/1, L/1, M/1, K_s/1, S/1
  kalman filter1/3(Y_error) -> MATLAB Function/1(err), Out2/1
  S/1 -> MATLAB Function/2(S)
  MATLAB Function/1(y) -> Out3/1

== system kalman_estimate_MM/HKF4 ==
  In2 : Inport
  In3 : Inport  Port=2
  In4 : Inport  Port=3
  x_obem : Inport  Port=4
  y_obem : Inport  Port=5
  A : sharedschedule/Interpolate Matrix(x)   matrix=piece.A  aMode=aMode
      settings: SourceProductName=Aerospace Blockset  SourceProductBaseCode=AE
  B : sharedschedule/Interpolate Matrix(x)   matrix=piece.B  aMode=aMode
      settings: SourceProductName=Aerospace Blockset  SourceProductBaseCode=AE
  C : sharedschedule/Interpolate Matrix(x)   matrix=piece.C  aMode=aMode
      settings: SourceProductName=Aerospace Blockset  SourceProductBaseCode=AE
  D : sharedschedule/Interpolate Matrix(x)   matrix=piece.D  aMode=aMode
      settings: SourceProductName=Aerospace Blockset  SourceProductBaseCode=AE
  K_s : sharedschedule/Interpolate Matrix(x)   matrix=piece.K_s  aMode=aMode
      settings: SourceProductName=Aerospace Blockset  SourceProductBaseCode=AE
  L : sharedschedule/Interpolate Matrix(x)   matrix=piece.L  aMode=aMode
      settings: SourceProductName=Aerospace Blockset  SourceProductBaseCode=AE
  M : sharedschedule/Interpolate Matrix(x)   matrix=piece.M  aMode=aMode
      settings: SourceProductName=Aerospace Blockset  SourceProductBaseCode=AE
  MATLAB Function : MATLAB Function  TreatAsAtomicUnit=on
  Minus5 : Sum  Inputs=+-
  Prelookup : PreLookup  BreakpointsData=piece.Nl  BreakpointObject=Nl  ExtrapMethod=Linear  UseLastBreakpoint=on  DiagnosticForOutOfRangeInput=Warning
  S : sharedschedule/Interpolate Matrix(x)   matrix=piece.S_s  aMode=aMode
      settings: SourceProductName=Aerospace Blockset  SourceProductBaseCode=AE
  Selector : Selector  InputPortWidth=2  IndexOptions=Index vector (dialog)  Indices=[1]  OutputSizes=1
  kalman filter1 : Subsystem
  steadyOutput : sharedschedule/Interpolate Matrix(x)   matrix=piece.steadyOutput  aMode=aMode
      settings: SourceProductName=Aerospace Blockset  SourceProductBaseCode=AE
  steadyState : sharedschedule/Interpolate Matrix(x)   matrix=piece.steadyState  aMode=aMode
      settings: SourceProductName=Aerospace Blockset  SourceProductBaseCode=AE
  steadyinput : sharedschedule/Interpolate Matrix(x)   matrix=piece.steadyInput  aMode=aMode
      settings: SourceProductName=Aerospace Blockset  SourceProductBaseCode=AE
  Out1 : Outport
  Out2 : Outport  Port=2
  Out3 : Outport  Port=3
  wires:
  Prelookup/1 -> S/1, K_s/1, M/1, L/1, steadyState/1, steadyinput/1, steadyOutput/1, D/1, C/1, B/1, A/1
  In4/1 -> kalman filter1/9(P)
  Prelookup/2 -> A/2, steadyState/2, S/2, K_s/2, M/2, L/2, steadyinput/2, steadyOutput/2, D/2, C/2, B/2
  Selector/1 -> Prelookup/1
  L/1 -> kalman filter1/7(L)
  C/1 -> kalman filter1/2(C)
  Minus5/1 -> kalman filter1/5(Y)
  kalman filter1/2(Y_es) -> Out1/1
  kalman filter1/1(X_es) -> Selector/1
  K_s/1 -> kalman filter1/3(K)
  A/1 -> kalman filter1/1(A)
  M/1 -> kalman filter1/8(M)
  In3/1 -> kalman filter1/4(x0)
  In2/1 -> Minus5/1
  y_obem/1 -> Minus5/2
  x_obem/1 -> kalman filter1/6(Xtrim)
  MATLAB Function/1(y) -> Out3/1
  kalman filter1/3(Y_error) -> MATLAB Function/1(err), Out2/1
  S/1 -> MATLAB Function/2(S)

== system kalman_estimate_MM/HKF5 ==
  In2 : Inport
  In3 : Inport  Port=2
  In4 : Inport  Port=3
  x_obem : Inport  Port=4
  y_obem : Inport  Port=5
  A : sharedschedule/Interpolate Matrix(x)   matrix=piece.A  aMode=aMode
      settings: SourceProductName=Aerospace Blockset  SourceProductBaseCode=AE
  B : sharedschedule/Interpolate Matrix(x)   matrix=piece.B  aMode=aMode
      settings: SourceProductName=Aerospace Blockset  SourceProductBaseCode=AE
  C : sharedschedule/Interpolate Matrix(x)   matrix=piece.C  aMode=aMode
      settings: SourceProductName=Aerospace Blockset  SourceProductBaseCode=AE
  D : sharedschedule/Interpolate Matrix(x)   matrix=piece.D  aMode=aMode
      settings: SourceProductName=Aerospace Blockset  SourceProductBaseCode=AE
  K_s : sharedschedule/Interpolate Matrix(x)   matrix=piece.K_s  aMode=aMode
      settings: SourceProductName=Aerospace Blockset  SourceProductBaseCode=AE
  L : sharedschedule/Interpolate Matrix(x)   matrix=piece.L  aMode=aMode
      settings: SourceProductName=Aerospace Blockset  SourceProductBaseCode=AE
  M : sharedschedule/Interpolate Matrix(x)   matrix=piece.M  aMode=aMode
      settings: SourceProductName=Aerospace Blockset  SourceProductBaseCode=AE
  MATLAB Function : MATLAB Function  TreatAsAtomicUnit=on
  Minus5 : Sum  Inputs=+-
  Prelookup : PreLookup  BreakpointsData=piece.Nl  BreakpointObject=Nl  ExtrapMethod=Linear  UseLastBreakpoint=on  DiagnosticForOutOfRangeInput=Warning
  S : sharedschedule/Interpolate Matrix(x)   matrix=piece.S_s  aMode=aMode
      settings: SourceProductName=Aerospace Blockset  SourceProductBaseCode=AE
  Selector : Selector  InputPortWidth=2  IndexOptions=Index vector (dialog)  Indices=[1]  OutputSizes=1
  kalman filter1 : Subsystem
  steadyOutput : sharedschedule/Interpolate Matrix(x)   matrix=piece.steadyOutput  aMode=aMode
      settings: SourceProductName=Aerospace Blockset  SourceProductBaseCode=AE
  steadyState : sharedschedule/Interpolate Matrix(x)   matrix=piece.steadyState  aMode=aMode
      settings: SourceProductName=Aerospace Blockset  SourceProductBaseCode=AE
  steadyinput : sharedschedule/Interpolate Matrix(x)   matrix=piece.steadyInput  aMode=aMode
      settings: SourceProductName=Aerospace Blockset  SourceProductBaseCode=AE
  Out1 : Outport
  Out2 : Outport  Port=2
  Out3 : Outport  Port=3
  wires:
  x_obem/1 -> Selector/1, kalman filter1/6(Xtrim)
  y_obem/1 -> Minus5/2
  In2/1 -> Minus5/1
  In3/1 -> kalman filter1/4(x0)
  M/1 -> kalman filter1/8(M)
  A/1 -> kalman filter1/1(A)
  K_s/1 -> kalman filter1/3(K)
  kalman filter1/2(Y_es) -> Out1/1
  Minus5/1 -> kalman filter1/5(Y)
  C/1 -> kalman filter1/2(C)
  L/1 -> kalman filter1/7(L)
  Selector/1 -> Prelookup/1
  Prelookup/2 -> B/2, C/2, D/2, steadyOutput/2, steadyinput/2, L/2, M/2, K_s/2, S/2, steadyState/2, A/2
  In4/1 -> kalman filter1/9(P)
  Prelookup/1 -> A/1, B/1, C/1, D/1, steadyOutput/1, steadyinput/1, steadyState/1, L/1, M/1, K_s/1, S/1
  MATLAB Function/1(y) -> Out3/1
  kalman filter1/3(Y_error) -> MATLAB Function/1(err), Out2/1
  S/1 -> MATLAB Function/2(S)

== system kalman_estimate_MM/HKF6 ==
  In2 : Inport
  In3 : Inport  Port=2
  In4 : Inport  Port=3
  x_obem : Inport  Port=4
  y_obem : Inport  Port=5
  A : sharedschedule/Interpolate Matrix(x)   matrix=piece.A  aMode=aMode
      settings: SourceProductName=Aerospace Blockset  SourceProductBaseCode=AE
  B : sharedschedule/Interpolate Matrix(x)   matrix=piece.B  aMode=aMode
      settings: SourceProductName=Aerospace Blockset  SourceProductBaseCode=AE
  C : sharedschedule/Interpolate Matrix(x)   matrix=piece.C  aMode=aMode
      settings: SourceProductName=Aerospace Blockset  SourceProductBaseCode=AE
  D : sharedschedule/Interpolate Matrix(x)   matrix=piece.D  aMode=aMode
      settings: SourceProductName=Aerospace Blockset  SourceProductBaseCode=AE
  K_s : sharedschedule/Interpolate Matrix(x)   matrix=piece.K_s  aMode=aMode
      settings: SourceProductName=Aerospace Blockset  SourceProductBaseCode=AE
  L : sharedschedule/Interpolate Matrix(x)   matrix=piece.L  aMode=aMode
      settings: SourceProductName=Aerospace Blockset  SourceProductBaseCode=AE
  M : sharedschedule/Interpolate Matrix(x)   matrix=piece.M  aMode=aMode
      settings: SourceProductName=Aerospace Blockset  SourceProductBaseCode=AE
  MATLAB Function : MATLAB Function  TreatAsAtomicUnit=on
  Minus5 : Sum  Inputs=+-
  Prelookup : PreLookup  BreakpointsData=piece.Nl  BreakpointObject=Nl  ExtrapMethod=Linear  UseLastBreakpoint=on  DiagnosticForOutOfRangeInput=Warning
  S : sharedschedule/Interpolate Matrix(x)   matrix=piece.S_s  aMode=aMode
      settings: SourceProductName=Aerospace Blockset  SourceProductBaseCode=AE
  Selector : Selector  InputPortWidth=2  IndexOptions=Index vector (dialog)  Indices=[1]  OutputSizes=1
  kalman filter1 : Subsystem
  steadyOutput : sharedschedule/Interpolate Matrix(x)   matrix=piece.steadyOutput  aMode=aMode
      settings: SourceProductName=Aerospace Blockset  SourceProductBaseCode=AE
  steadyState : sharedschedule/Interpolate Matrix(x)   matrix=piece.steadyState  aMode=aMode
      settings: SourceProductName=Aerospace Blockset  SourceProductBaseCode=AE
  steadyinput : sharedschedule/Interpolate Matrix(x)   matrix=piece.steadyInput  aMode=aMode
      settings: SourceProductName=Aerospace Blockset  SourceProductBaseCode=AE
  Out1 : Outport
  Out2 : Outport  Port=2
  Out3 : Outport  Port=3
  wires:
  Prelookup/1 -> S/1, K_s/1, M/1, L/1, steadyState/1, steadyinput/1, steadyOutput/1, D/1, C/1, B/1, A/1
  In4/1 -> kalman filter1/9(P)
  Prelookup/2 -> A/2, steadyState/2, S/2, K_s/2, M/2, L/2, steadyinput/2, steadyOutput/2, D/2, C/2, B/2
  Selector/1 -> Prelookup/1
  L/1 -> kalman filter1/7(L)
  C/1 -> kalman filter1/2(C)
  Minus5/1 -> kalman filter1/5(Y)
  kalman filter1/2(Y_es) -> Out1/1
  kalman filter1/1(X_es) -> Selector/1
  K_s/1 -> kalman filter1/3(K)
  A/1 -> kalman filter1/1(A)
  M/1 -> kalman filter1/8(M)
  In3/1 -> kalman filter1/4(x0)
  In2/1 -> Minus5/1
  y_obem/1 -> Minus5/2
  x_obem/1 -> kalman filter1/6(Xtrim)
  MATLAB Function/1(y) -> Out3/1
  kalman filter1/3(Y_error) -> MATLAB Function/1(err), Out2/1
  S/1 -> MATLAB Function/2(S)

== system kalman_estimate_MM/HKF7 ==
  In2 : Inport
  In3 : Inport  Port=2
  In4 : Inport  Port=3
  x_obem : Inport  Port=4
  y_obem : Inport  Port=5
  A : sharedschedule/Interpolate Matrix(x)   matrix=piece.A  aMode=aMode
      settings: SourceProductName=Aerospace Blockset  SourceProductBaseCode=AE
  B : sharedschedule/Interpolate Matrix(x)   matrix=piece.B  aMode=aMode
      settings: SourceProductName=Aerospace Blockset  SourceProductBaseCode=AE
  C : sharedschedule/Interpolate Matrix(x)   matrix=piece.C  aMode=aMode
      settings: SourceProductName=Aerospace Blockset  SourceProductBaseCode=AE
  D : sharedschedule/Interpolate Matrix(x)   matrix=piece.D  aMode=aMode
      settings: SourceProductName=Aerospace Blockset  SourceProductBaseCode=AE
  K_s : sharedschedule/Interpolate Matrix(x)   matrix=piece.K_s  aMode=aMode
      settings: SourceProductName=Aerospace Blockset  SourceProductBaseCode=AE
  L : sharedschedule/Interpolate Matrix(x)   matrix=piece.L  aMode=aMode
      settings: SourceProductName=Aerospace Blockset  SourceProductBaseCode=AE
  M : sharedschedule/Interpolate Matrix(x)   matrix=piece.M  aMode=aMode
      settings: SourceProductName=Aerospace Blockset  SourceProductBaseCode=AE
  MATLAB Function : MATLAB Function  TreatAsAtomicUnit=on
  Minus5 : Sum  Inputs=+-
  Prelookup : PreLookup  BreakpointsData=piece.Nl  BreakpointObject=Nl  ExtrapMethod=Linear  UseLastBreakpoint=on  DiagnosticForOutOfRangeInput=Warning
  S : sharedschedule/Interpolate Matrix(x)   matrix=piece.S_s  aMode=aMode
      settings: SourceProductName=Aerospace Blockset  SourceProductBaseCode=AE
  Selector : Selector  InputPortWidth=2  IndexOptions=Index vector (dialog)  Indices=[1]  OutputSizes=1
  kalman filter1 : Subsystem
  steadyOutput : sharedschedule/Interpolate Matrix(x)   matrix=piece.steadyOutput  aMode=aMode
      settings: SourceProductName=Aerospace Blockset  SourceProductBaseCode=AE
  steadyState : sharedschedule/Interpolate Matrix(x)   matrix=piece.steadyState  aMode=aMode
      settings: SourceProductName=Aerospace Blockset  SourceProductBaseCode=AE
  steadyinput : sharedschedule/Interpolate Matrix(x)   matrix=piece.steadyInput  aMode=aMode
      settings: SourceProductName=Aerospace Blockset  SourceProductBaseCode=AE
  Out1 : Outport
  Out2 : Outport  Port=2
  Out3 : Outport  Port=3
  wires:
  x_obem/1 -> kalman filter1/6(Xtrim)
  y_obem/1 -> Minus5/2
  In2/1 -> Minus5/1
  In3/1 -> kalman filter1/4(x0)
  M/1 -> kalman filter1/8(M)
  A/1 -> kalman filter1/1(A)
  K_s/1 -> kalman filter1/3(K)
  kalman filter1/1(X_es) -> Selector/1
  kalman filter1/2(Y_es) -> Out1/1
  Minus5/1 -> kalman filter1/5(Y)
  C/1 -> kalman filter1/2(C)
  L/1 -> kalman filter1/7(L)
  Selector/1 -> Prelookup/1
  Prelookup/2 -> B/2, C/2, D/2, steadyOutput/2, steadyinput/2, L/2, M/2, K_s/2, S/2, steadyState/2, A/2
  In4/1 -> kalman filter1/9(P)
  Prelookup/1 -> A/1, B/1, C/1, D/1, steadyOutput/1, steadyinput/1, steadyState/1, L/1, M/1, K_s/1, S/1
  MATLAB Function/1(y) -> Out3/1
  kalman filter1/3(Y_error) -> MATLAB Function/1(err), Out2/1
  S/1 -> MATLAB Function/2(S)
